simulink model "prob7_week1"  (R2020b)
settings: Solver=VariableStepAuto  StartTime=0.0  StopTime=10.0  RelTol=1e-3
settings Model: Creator=Pulkit Khandelwal  LastModifiedBy=Pulkit Khandelwal

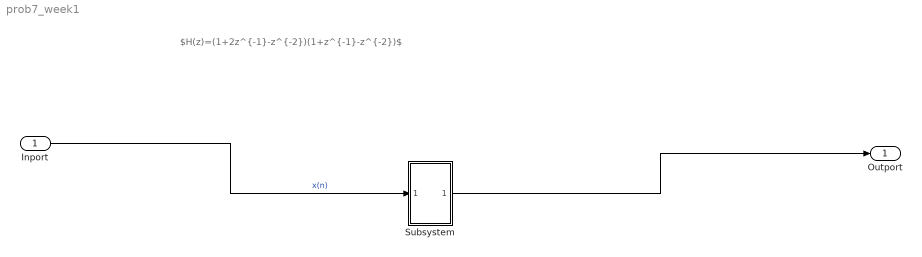
== system prob7_week1 ==
  note: $H(z)=(1+2z^{-1}-z^{-2})(1+z^{-1}-z^{-2})$
  Inport : Inport  OutDataTypeStr=double  PortDimensions=1  SampleTime=[0.20000000000000001,0]
  Subsystem : Subsystem  TreatAsAtomicUnit=on
  Outport : Outport  OutDataTypeStr=double  PortDimensions=1  SampleTime=[0.20000000000000001,0]
  wires:
  Inport/1 -> Subsystem/1(x(n))  "x(n)"
  Subsystem/1(y(n)) -> Outport/1

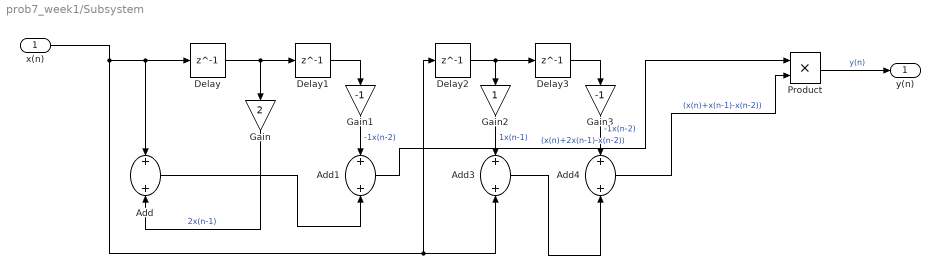
== system prob7_week1/Subsystem ==
  x(n) : Inport
  Add{,1,3..4} (4 alike) : Sum
  Delay{,1..3} (4 alike) : Delay  DelayLength=1
  Gain : Gain  Gain=2
  Gain1 : Gain  Gain=-1
  Gain2 : Gain
  Gain3 : Gain  Gain=-1
  Product : Product
  y(n) : Outport
  wires:
  Gain2/1 -> Add3/1  "1x(n-1)"
  Add3/1 -> Add4/2
  Gain/1 -> Add/2  "2x(n-1)"
  Add1/1 -> Product/1  "(x(n)+2x(n-1)-x(n-2))"
  x(n)/1 -> Add/1, Delay/1, Add3/2, Delay2/1
  Delay/1 -> Gain/1, Delay1/1
  Delay3/1 -> Gain3/1
  Delay1/1 -> Gain1/1
  Add4/1 -> Product/2  "(x(n)+x(n-1)-x(n-2))"
  Gain1/1 -> Add1/1  "-1x(n-2)"
  Add/1 -> Add1/2
  Gain3/1 -> Add4/1  "-1x(n-2)"
  Delay2/1 -> Gain2/1, Delay3/1
  Product/1 -> y(n)/1  "y(n)"
